simulink model "main_RI_LIEKF_GNSSOutrage"  (R2023a)
settings: Solver=FixedStepAuto  StartTime=0.0  StopTime=220  FixedStep=0.01  RelTol=1e-3
InitFcn:
  | initNavigation0612_AOA;
values from neighbouring files (symbols this model uses):
  CF_enable = 0    [initNavigation.m]
  dt = 0.01    [initNavigation.m]
  dtDelay = -0.03    [initNavigation.m]
  g0 = 9.795    [initNavigation.m]
  gam0_rad = 0/57.3    (= 0)    [initNavigation.m]
  GNSSoutragetime = 90    [initNavigation.m]
  H_sensor_type = 0    [initNavigation.m]
  KF_enable = 1    [initNavigation.m]
  P0 = diag([1*ones(3,1);0.01*ones(3,1);0.1*ones(3,1);0.001*ones(3,1);0.00001*ones(3,1)])    [initNavigation.m]
  P0_RIEKF = diag([1*ones(3,1);0.01*ones(3,1);0.1*ones(3,1);0.001*ones(3,1);0.00001*ones(3,1);      0.01*ones(3,1);[0;2;2]/57.3;[0.1;0.1;0.1]])^2    [initNavigation.m]
  pd0 = 0    [initNavigation.m]
  pe0 = 0    [initNavigation.m]
  phi0_rad = 0/57.3    (= 0)    [initNavigation.m]
  pn0 = 0    [initNavigation.m]
  psi = -178    [initNavigation.m]
  psi0_rad = 0/57.3    (= 0)    [initNavigation.m]
  state_dim = 24    [initNavigation.m]
  Time = 0:0.01:(size(traindata.AttackAngle,1) - 1)*0.01    [NNLiftCoefficientFit.m]
  vd0 = 0    [initNavigation.m]
  ve0 = 0    [initNavigation.m]
  vn0 = 0    [initNavigation.m]
undefined symbols (not defined in the file or in its folder): DiscIntNeverNeededParam, Discrete, INS_CONST, INS_EXPORT, INS_PARAM, magnitude, p, param, pInitialization, sys
libraries: simulink_extras x94, simulink x82, dspstat3 x70, sharedtransform x60, ctrlSharedLib x36, sharedTrackingLibrary x22, matrix_library x15, FMT_Model_Lib x13, deeplib x8, dspsolvers x4, vrlib x4, aerolibconvert2 x1
(part 25 of 28)

== matlab function main_RI_LIEKF_GNSSOutrage/State estimation/RI EKF_AOA_direct/Error State Kalman Filter/bak/Simulink Function - State Transition Jacobian/Cal Phi1/MATLAB Function1 ==
  data: vn input; Phi output; pn input; Rbn input; dt input
function Phi = fcn(vn,pn, Rbn,dt)
    
    %{
    F.block(0, 0, 3, 3) = exp_so3(-w_hat * dt);
        F.block(0, 9, 3, 3).noalias() = -exp_so3(-w_hat * dt) * Jr_so3(-w_hat * dt) * dt;
        F.block(9, 9, 3, 3).setIdentity();
        F.block(6, 0, 3, 3).noalias() = -R_Gtoi.transpose() * skew_x(a_hat * dt);
        F.block(6, 6, 3, 3).setIdentity();
        F.block(6, 12, 3, 3) = -R_Gtoi.transpose() * dt;
        F.block(12, 12, 3, 3).setIdentity();
        F.block(3, 0, 3, 3).noalias() = -0.5 * R_Gtoi.transpose() * skew_x(a_hat * dt * dt);
        F.block(3, 6, 3, 3) = Eigen::Matrix3d::Identity() * dt;
        F.block(3, 12, 3, 3) = -0.5 * R_Gtoi.transpose() * dt * dt;
        F.block(3, 3, 3, 3).setIdentity();
        Eigen::Matrix<double, 15, 12> G = Eigen::Matrix<double, 15, 12>::Zero();
    %}
    %
    %
    %F = [0_33         0_33  0_33   -Rbn          0_33]
    %    [skew(gn)     0_33  0_33  -skew(vn)Rbn   -Rbn]
    %    [0.5*skew(gn) I_33  0_33  -skew(pn)Rbn   -Rbn]
    %    [         0_69                  I66          ]
    Phi = zeros(15,15);
    g0 = 9.79;
    gn = [0;0;-g0];
    F  = zeros(15,15);
    F(1:3,10:12) = -Rbn;
    F(4:6,1:3)   = skewMat(gn);
    F(4:6,10:12) = -skewMat(vn)*Rbn;
    F(4:6,13:15) = -Rbn;
    F(7:9,4:6)   = eye(3);
    F(7:9,1:3)   = 0.5*skewMat(gn) * dt;
    F(7:9,10:12) = -skewMat(pn)*Rbn;
    F(7:9,13:15) = -Rbn;
    %F(10:15,10:15) = eye(6);
    Phi = eye(15) + F * dt;

end

== matlab function main_RI_LIEKF_GNSSOutrage/State estimation/RI EKF_AOA_direct/Error State Kalman Filter/bak/Simulink Function - State Transition Jacobian/MATLAB Function1 ==
  data: Rbn input; G output; vn input; pn input; dt input
function G = fcn(Rbn, vn,pn, dt)
    % G.block(0, 0, 3, 3) = -exp_so3(-w_hat * dt) * Jr_so3(-w_hat * dt) * dt;
    %    G.block(6, 3, 3, 3) = -R_Gtoi.transpose() * dt;
    %    G.block(3, 3, 3, 3) = -0.5 * R_Gtoi.transpose() * dt * dt;
    %    G.block(9, 6, 3, 3).setIdentity();
    %    G.block(12, 9, 3, 3).setIdentity();

    G = zeros(15,12);
    % G(1:3,1:3) = -  Rbn * dt;
    % G(4:6,1:3) = -skewMat(vn)*Rbn* dt;
    % G(4:6,4:6) =  - Rbn;
    % G(7:9,1:3) = -skewMat(pn)*Rbn * dt;
    % G(7:9,4:6) =  - Rbn;
    % G(10:12,7:9) = eye(3)*dt;
    % G(13:15,10:12) = eye(3)*dt;
    G(1:3,1:3) =  - Rbn * dt;
    G(4:6,1:3) = -skewMat(vn)*Rbn * dt;
    G(4:6,4:6) =  - Rbn* dt;
    G(7:9,1:3) = -skewMat(pn)*Rbn * dt;
    G(7:9,4:6) =  - Rbn* dt;
    G(10:12,7:9) = eye(3) ;
    G(13:15,10:12) = eye(3) ;
    
    %G = G*double(dt);
end

== matlab function main_RI_LIEKF_GNSSOutrage/State estimation/RI EKF_AOA_direct/INS propogation/AOA//SA//Vwind update/Subsystem/MATLAB Function ==
  data: u input; Rab output
function Rab = fcn(u)
    Rab = zeros(3,3);
        ca = cos(u(2));
        sa = sin(u(2));
        cb = cos(u(3));
        sb = sin(u(3));
    Rab = double([ca * cb,-ca * sb, -sa;
        sb, cb, 0;
        sa * cb, -sa * sb, ca;]);
end

== matlab function main_RI_LIEKF_GNSSOutrage/State estimation/RI EKF_AOA_direct/INS propogation/AOA//SA//Vwind update/Subsystem/MATLAB Function2 ==
  data: delta input; Rbn_correct output double size=[3,3]; Rbn input
function Rbn_correct = fcn(delta, Rbn)
    delta(1) = 0;
    Rbn_correct = zeros(3,3);
     %Rbn_correct = exp_so3(delta)* Rbn;
    Rbn_correct =double(( eye(3) + skewMat(delta))* Rbn);
end

== matlab function main_RI_LIEKF_GNSSOutrage/State estimation/RI EKF_AOA_direct/INS propogation/AOA//SA//Vwind update/Subsystem/Subsystem1/LSTM predict/MATLAB Function5 ==
  data: X input; X_nYPred output
function X_nYPred = LSTMnet(X)
    sig_X = [0.1167;0.1277;0.0579];
    sig_Y = 0.0451;
    mu_X = [0.0587;0.5185;-0.0515];
    mu_Y = 0.1011;
    X_norm = (X - mu_X) ./ sig_X;
    persistent X_nYPredorm_store;
    if isempty(X_nYPredorm_store)
        X_nYPredorm_store = zeros(1000,3);
    end

    X_nYPredorm_store = [X_nYPredorm_store(2:end,:);X_norm'];
    %[~,YPred_seq] = predictAndUpdateState(net.net,X_nYPredorm_store);
     X_nYPred = single(X_nYPredorm_store);
    % YPred_seq = predict(net.net,X_nYPredorm_store');
    % YPred_test = YPred_seq(end);
    % YPred_test = double(YPred_test* sig_Y + mu_Y)*57.3;

end

== matlab function main_RI_LIEKF_GNSSOutrage/State estimation/RI EKF_AOA_direct/INS propogation/AOA//SA//Vwind update/Subsystem/Subsystem1/LSTM predict/MATLAB Function6 ==
  data: YPred_test input; YPred_test_out output
function YPred_test_out = LSTMnet(YPred_test)
    sig_X = [0.1167;0.1277;0.0579];
    sig_Y = 0.0451;
    mu_X = [0.0587;0.5185;-0.0515];
    mu_Y = 0.1011;
    YPred_test_out = YPred_test(end);
    YPred_test_out = single(YPred_test_out* sig_Y + mu_Y)*57.3;

end

== matlab function main_RI_LIEKF_GNSSOutrage/State estimation/RI EKF_AOA_direct/INS propogation/AOA//SA//Vwind update/Subsystem/Subsystem1/LSTM predict1/MATLAB Function5 ==
  data: X input; X_nYPred output
function X_nYPred = LSTMnet(X)
    sig_X = [0.2380; 0.1523 ;0.0429;0.1379];
    sig_Y = 0.0690;
    mu_X = [0.0068;-0.0055;-0.0070;-0.0450];
    mu_Y = -0.0228;
    X_norm = (X - mu_X) ./ sig_X;
    persistent X_nYPredorm_store;
    if isempty(X_nYPredorm_store)
        X_nYPredorm_store = zeros(1000,4);
    end

    X_nYPredorm_store = [X_nYPredorm_store(2:end,:);X_norm'];
    %[~,YPred_seq] = predictAndUpdateState(net.net,X_nYPredorm_store);
     X_nYPred = single(X_nYPredorm_store);
    % YPred_seq = predict(net.net,X_nYPredorm_store');
    % YPred_test = YPred_seq(end);
    % YPred_test = double(YPred_test* sig_Y + mu_Y)*57.3;

end

== matlab function main_RI_LIEKF_GNSSOutrage/State estimation/RI EKF_AOA_direct/INS propogation/AOA//SA//Vwind update/Subsystem/Subsystem1/LSTM predict1/MATLAB Function6 ==
  data: YPred_test input; YPred_test_out output
function YPred_test_out = LSTMnet(YPred_test)
    sig_X = [0.2380; 0.1523 ;0.0429;0.1379];
    sig_Y = 0.0690;
    mu_X = [0.0068;-0.0055;-0.0070;-0.0450];
    mu_Y = -0.0228;
    YPred_test_out = YPred_test(end);
    YPred_test_out = single(YPred_test_out* sig_Y + mu_Y)*57.3;

end

== matlab function main_RI_LIEKF_GNSSOutrage/State estimation/RI EKF_AOA_direct/INS propogation/AOA//SA//Vwind update/Subsystem/Subsystem1/MATLAB Function1 ==
  data: axyz input; Cl output; TAS input; alpha input
function Cl = fcn(axyz, TAS,alpha)
ax = axyz(1);
az = axyz(3);
mess = 6.9;
g = 9.79;
rou = 1.225;
a = 1.4;
b = 0.36;
S = a*b;

q = 0.5 * rou * TAS^2;

azs = -ax * sin(alpha) + az * cos(alpha);
Cl = -mess * azs / (q * S);
end

== matlab function main_RI_LIEKF_GNSSOutrage/Sensor_Data_Process/IMU_Data_Process/accl_preprocessing2/MATLAB Function3 ==
  data: curr_input input; curr_output output single; sample_freq input; cutoff_freq input
function curr_output = second_LPF_Butter_x(curr_input,sample_freq,cutoff_freq)
   persistent input_x;
   persistent output_x;

   if isempty(input_x)
       input_x = [0;0;0];
   end
   
   if isempty(output_x)
       output_x = [0;0;0];
   end
    B = [0,0,0];
    A = [0,0,0];
    M_PI_F = 3.1415926;
	fr = sample_freq / cutoff_freq;
	ohm = tan( M_PI_F / fr );
	c = 1.0 + 2.0 * cos( M_PI_F / 4.0 ) * ohm + ohm * ohm;
	B(1) = ohm * ohm / c;
	B(2) = 2.0 * B(1);
	B(3) = B(1);
	A(1) = 2.0 * ( ohm * ohm - 1.0) / c;
	A(2) = (1.0 - 2.0 * cos( M_PI_F / 4.0 ) * ohm + ohm * ohm) / c;
	%/*获取最新输入*/
	input_x(3) = curr_input;
	%/* Butterworth */
	output_x(3) =B(1) * input_x(3) + B(2) * input_x(2) +B(3) * input_x(1) - A(1) * output_x(2) - A(2) * output_x(1);
	curr_output = single(output_x(3));
   % /* 输入序列保存 */
	input_x(1) = input_x(2);
	input_x(2) = input_x(3);
	%/*输出序列保存 */
	output_x(1) = output_x(2);
	output_x(2) = output_x(3);

== matlab function main_RI_LIEKF_GNSSOutrage/State estimation/RI EKF_AOA_direct/INS propogation/AOA//SA//Vwind update/Subsystem/Subsystem1/MATLAB Function3 ==
  data: axyz input; Cy output; TAS input; alpha input; beta input
function Cy = fcn(axyz, TAS,alpha,beta)
ax = axyz(1);
ay = axyz(2);
az = axyz(3);

mess = 6.9;
g = 9.79;
rou = 1.225;
a = 1.4;
b = 0.36;
S = a*b;

q = 0.5 * rou * TAS^2;
ays = -ax .* cos(alpha).*sin(beta) + ay .* cos(beta) - az .* sin(alpha).* sin(beta);
% azs = -ax * sin(alpha) + az * cos(alpha);
Cy = mess * ays / (q * S);
end

== matlab function main_RI_LIEKF_GNSSOutrage/State estimation/RI EKF_AOA_direct/INS propogation/AOA//SA//Vwind update/Subsystem/Subsystem1/MATLAB Function4 ==
  data: u input; CalculatedAttackAngleFiltered output
function CalculatedAttackAngleFiltered = fcn(u)
PitchRate = u(1);
cl = u(2);
ElevatorAngle = u(3);

coefficients_filtered = [0.0236, -0.4283, -0.0765, -0.0898];

    
CalculatedAttackAngleFiltered = (cl - ...
    coefficients_filtered(1) - ...
    coefficients_filtered(3) * PitchRate - ...
    coefficients_filtered(4) * ElevatorAngle) / coefficients_filtered(2);


end

== matlab function main_RI_LIEKF_GNSSOutrage/State estimation/RI EKF_AOA_direct/INS propogation/att update/MATLAB Function ==
  data: Rbn_k_1 input; Rbn output; w input; dt input
function Rbn = fcn(Rbn_k_1, w, dt)
    Rbn =  Rbn_k_1 * exp_so3( w * dt);
end

== matlab function main_RI_LIEKF_GNSSOutrage/State estimation/RI EKF_AOA_direct/INS propogation/att update/MATLAB Function2 ==
  data: delta input; Rbn_correct output single size=[3,3]; Rbn input
function Rbn_correct = fcn(delta, Rbn)
    Rbn_correct = zeros(3,3);
     Rbn_correct = exp_so3(delta)* Rbn;
    %Rbn_correct =( eye(3) + skewMat(delta))* Rbn;
end

== matlab function main_RI_LIEKF_GNSSOutrage/State estimation/RI EKF_AOA_direct/INS propogation/vel//pos update/pos update/MATLAB Function ==
  data: dtheta input; pos_correct output single; KFState_dp input; pos input
function pos_correct = fcn(dtheta, KFState_dp, pos)
    
     pos_correct =  KFState_dp + exp_so3(dtheta)*pos;
    %pos_correct = pos + KFState_dp - skewMat(pos)*dtheta;
    
end

== matlab function main_RI_LIEKF_GNSSOutrage/State estimation/RI EKF_AOA_direct/INS propogation/vel//pos update/vel update/MATLAB Function ==
  data: dtheta input; vel_correct output single; KFState_dv input; vel input
function vel_correct = fcn(dtheta, KFState_dv, vel)
    
     vel_correct =  KFState_dv + exp_so3( dtheta)*vel;
    %vel_correct =  vel + KFState_dv - skewMat(vel)*dtheta;
end

== matlab function main_RI_LIEKF_GNSSOutrage/State estimation/LI EKF2/Error State Kalman Filter/Extended Kalman Filter1/Correct1/IGG_check/MATLAB Function ==
  data: err input; w output; k0 input; k1 input; zk0 input; zk1 input
function w = fcn(err,k0,k1,zk0,zk1)
    err = abs(err);  w = err;
    for k=1:2
        if err(k)<=k0,    w(k)=1;
        elseif err(k)>k1, w(k)=0;
        else,             w(k)=k0/err(k);  
        end
    end
        if err(3)<=zk0,    w(3)=1;
        elseif err(3)>zk1, w(3)=0;
        else,             w(3)=zk0/err(3);  
        end
end

== matlab function main_RI_LIEKF_GNSSOutrage/State estimation/LI EKF2/Error State Kalman Filter/Extended Kalman Filter1/Output/MATLAB Function ==
  data: S input; P output
function P = fcn(S)
    
    % Get back Covariance from Square-root Covariance
    P = S*S';
    
end

== matlab function main_RI_LIEKF_GNSSOutrage/State estimation/LI EKF2/Error State Kalman Filter/Extended Kalman Filter1/Predict/Predict ==
  settings: updateMethod=DISCRETE  sampleTime=SampleTime
  data: x input; xNew output; P input; Q input; uState input; unused input; P output; pS parameter
function [xNew,P] = fcn(x,P,Q,uState,~,pS)
% ekfCorrect Prediction step for EKF
%
%   Copyright 2016-2021 The MathWorks, Inc.

%#codegen

% If process noise is time-varying then compute square-root
% factorization.
if pS.HasTimeVaryingQ
   Q = matlabshared.tracking.internal.svdPSD(Q);
end

% Construct fcn handles
if pS.IsSimulinkFcn
    StateTransitionJacobianFcnH_SL = str2func(pS.FcnName);
    if pS.HasAdditiveNoise
        StateTransitionFcnH = @(fState)StateTransitionJacobianFcnH_SL(fState);
    else
        StateTransitionFcnH = @(fState,fProcNoise)StateTransitionJacobianFcnH_SL(fState,fProcNoise);
    end
else
    StateTransitionFcnH = str2func(pS.FcnName);
end
if pS.HasJacobian
    if pS.IsSimulinkFcn
        StateTransitionJacobianFcnH_SL = str2func(pS.JacobianFcnName);
        if pS.HasAdditiveNoise
            StateTransitionJacobianFcnH = @(fState)StateTransitionJacobianFcnH_SL(fState);
        else
            StateTransitionJacobianFcnH = @(fState,fProcNoise)StateTransitionJacobianFcnH_SL(fState,fProcNoise);
        end
    else
        StateTransitionJacobianFcnH = str2func(pS.JacobianFcnName);
    end
else
    StateTransitionJacobianFcnH = [];
end

switch pS.NumberOfExtraArgumentInports
    case 0
        extraArgs = {};
    case 1
        extraArgs = {uState};
    otherwise
        assert(false);
end

% Check if dimensions and type of State and Jacobian are correct
if pS.HasAdditiveNoise
   % Additive noise
   
   % StateTransitionFcn
   xTry = StateTransitionFcnH(x, extraArgs{:});
   
   if pS.IsSimulinkFcn
      hasError = any(size(x) ~= size(xTry));
   else
      hasError = any(size(x) ~= size(xTry)) || ~isa(xTry, class(x));
   end
   
   coder.internal.errorIf(...
      hasError,...
      'shared_tracking:ExtendedKalmanFilter:StateNonMatchingSizeOrClass',...
      'StateTransitionFcn', 'State', numel(x));
   
   if pS.HasJacobian
      % Jacobian
      F = StateTransitionJacobianFcnH(x, extraArgs{:});
      % F needs to be square
      isSizeNotCorrect = ~all(size(F) == numel(x));
      
      if pS.IsSimulinkFcn
         hasError = isSizeNotCorrect;
      else
         hasError = isSizeNotCorrect || ~isa(F, class(x));
      end
      
      coder.internal.errorIf(...
         hasError,...
         'shared_tracking:ExtendedKalmanFilter:StateTransitionJacobianNonMatchingSizeOrClass',...
         'StateTransitionJacobianFcn', numel(x));
   end
else
   % Non-additive noise
   
   % StateTransitionFcn
   xTry = StateTransitionFcnH(x, zeros(size(Q,1),1,'like',x),extraArgs{:});
   
   if pS.IsSimulinkFcn
      hasError = any(size(x) ~= size(xTry));
   else
      hasError = any(size(x) ~= size(xTry)) || ~isa(xTry, class(x));
   end
   
   coder.internal.errorIf(...
      hasError,...
      'shared_tracking:ExtendedKalmanFilter:StateNonMatchingSizeOrClass',...
      'StateTransitionFcn', 'State', numel(x))
   
   if pS.HasJacobian
      % Jacobian
      F = StateTransitionJacobianFcnH(x, zeros(size(Q,1),1,'like',x),extraArgs{:});
      % F needs to be square
      isSizeNotCorrect = ~all(size(F) == numel(x));
      
      if pS.IsSimulinkFcn
         hasError = isSizeNotCorrect;
      else
         hasError = isSizeNotCorrect || ~isa(F, class(x));
      end
       
      coder.internal.errorIf(...
         hasError,...
         'shared_tracking:ExtendedKalmanFilter:StateTransitionJacobianNonMatchingSizeOrClass',...
         'StateTransitionJacobianFcn', numel(x));
   end
end

xNew = zeros(size(x),'like',x); %#ok<PREALL>

if pS.HasAdditiveNoise
    [xNew,P] = matlabshared.tracking.internal.EKFPredictorAdditive.predict(...
        Q,x,P,StateTransitionFcnH,StateTransitionJacobianFcnH,extraArgs{:});
else    
    [xNew,P] = matlabshared.tracking.internal.EKFPredictorNonAdditive.predict(...
        Q,x,P,StateTransitionFcnH,StateTransitionJacobianFcnH,extraArgs{:});
end
end

== matlab function main_RI_LIEKF_GNSSOutrage/State estimation/LI EKF2/Error State Kalman Filter/MATLAB Function ==
  data: u input; dp output size=3; dv output size=3; dtheta output size=3; da output size=3; dg output size=3; dm output size=3; dtheta_a output size=3; dv_wind output size=3
function [dp,dv,dtheta,da,dg,dm,dtheta_a,dv_wind] = fcn(u)
    dtheta = u(1:3);
    dv = u(4:6);
    dp = u(7:9);
    dg = u(10:12);
    da = u(13:15);
    dm = u(16:18);
    dtheta_a = u(19:21);
    dv_wind = u(22:24);
end

== matlab function main_RI_LIEKF_GNSSOutrage/Subsystem2/MATLAB Function1 ==
  data: x input; angleHeadingAB0to360 output
function angleHeadingAB0to360 = fcn(x)
 x = x -180;


    if  x >= 0 && x < 90           %第一象限，范围 [0,90)deg，0度应该会出现
        angleHeadingAB0to360  =   x;
    elseif x >= 90 && x < 180       %第二象限，范围 [90,180)deg
        angleHeadingAB0to360 = x;
    elseif x >= 180 && x < 270     %第三象限，范围 [180,270)deg，180度也应该会出现
        angleHeadingAB0to360 = - 360 + x;
    elseif x >= 270 && x < 360      %第四象限，范围 [270,360)deg
        angleHeadingAB0to360  = - 360+x;
    elseif x< 0 && x>-90 
        angleHeadingAB0to360  =   x;
    elseif x<= -90 && x>-180
        angleHeadingAB0to360  =   x;
    elseif x <= -180 && x >= -360
        angleHeadingAB0to360  =   x + 360;
    elseif x == 0 && x == 360 
        angleHeadingAB0to360 =single(0);
    else
         angleHeadingAB0to360  =   x;
    end
end

== matlab function main_RI_LIEKF_GNSSOutrage/State estimation/distribute CF/distribute CF/Correct/Attitude_Correction/Attitude_Correct/Subsystem2/MATLAB Function ==
  data: abs_v input; y output; gps_acc input
function y = fcn(abs_v,gps_acc)
if abs_v < 0.1
    y = double(zeros(3,1));
elseif abs_v  >= 0.1 && abs_v < 1
    y = double(0.7* gps_acc);
else
    y = double(1 * gps_acc);
end

== matlab function main_RI_LIEKF_GNSSOutrage/State estimation/distribute CF/distribute CF/Update/Attitude_Update/QuatMult1 ==
  data: quatA input; quatOut output single; quatB input
function quatOut = QuatMult(quatA,quatB)
% Calculate the following quaternion product quatA * quatB using the 
% standard identity 

quatOut = [quatA(1)*quatB(1)-quatA(2:4)'*quatB(2:4); quatA(1)*quatB(2:4) + quatB(1)*quatA(2:4) + cross(quatA(2:4),quatB(2:4))];

== matlab function main_RI_LIEKF_GNSSOutrage/State estimation/distribute CF/distribute CF/Update/Attitude_Update/rv2q ==
  data: rotVec input single; quaternion output single
% convert froma rotation vector in radians to a quaternion
function quaternion = RotToQuat(rotVec)

vecLength = sqrt(rotVec(1)^2 + rotVec(2)^2 + rotVec(3)^2);

if vecLength < 1e-6
  quaternion = single([1;0;0;0]);
else
  quaternion = single([cos(0.5*vecLength); rotVec/vecLength*sin(0.5*vecLength)]);
end

== matlab function main_RI_LIEKF_GNSSOutrage/State estimation/LI EKF2/Error State Kalman Filter/Simulink Function - GPS Measurements/MATLAB Function ==
  data: vn input; H output; pn input
function H = fcn(vn, pn)
    state_dim = 24;
    H = zeros(6,state_dim);
    % H(1:3,1:3) = skewMat(vn);
    % H(4:6,1:3) = skewMat(pn);
    H(1:6,4:9) = eye(6);
    %H = -H;
end

== matlab function main_RI_LIEKF_GNSSOutrage/State estimation/LI EKF2/Error State Kalman Filter/Simulink Function - GPS Measurements/MATLAB Function1 ==
  data: Rbn input; vn input; X_inv output; pn input
function X_inv = invX(Rbn, vn, pn)
    X_inv = zeros(5,5);
    Rnb = Rbn';
    X_inv(1:3,1:3) = Rnb;
    X_inv(1:3,4) = -Rnb * vn;
    X_inv(1:3,5) = -Rnb * pn;
    X_inv(4:5,4:5) = eye(2);
end

== matlab function main_RI_LIEKF_GNSSOutrage/State estimation/LI EKF2/Error State Kalman Filter/Simulink Function - GPS Measurements1/MATLAB Function ==
  data: vn input; H_baro output; pn input
function H_baro = fcn(vn, pn)
    state_dim = 24;
    H = zeros(6,state_dim);
    H(1:3,1:3) = skewMat(vn);
    H(4:6,1:3) = skewMat(pn);
    H(1:6,4:9) = eye(6);
    
    A = [0 0 0 0 0 1];
    H_baro = A * H;
end

== matlab function main_RI_LIEKF_GNSSOutrage/State estimation/LI EKF2/Error State Kalman Filter/Simulink Function - GPS Measurements2/MATLAB Function ==
  data: Rbn input; Magn input; H output; dtheta input
function H = fcn(Rbn, Magn, dtheta)
    state_dim = 24;
    H = zeros(3,state_dim);
    H(1:3,1:3) =  Rbn * skewMat(Magn);
    H(1:3,16:18) =  Rbn * skewMat(dtheta);
end

== matlab function main_RI_LIEKF_GNSSOutrage/State estimation/LI EKF2/Error State Kalman Filter/Simulink Function - GPS Measurements3/MATLAB Function ==
  data: Rbn input; Rab input; H output; vn input; v_wind input
function H = fcn(Rbn,Rab, vn,v_wind)
    state_dim = 24;
    A = Rab' * Rbn';
    H = zeros(3,state_dim);
   % H(1:3,1:3) =  - skewMat(vn - v_wind);
   % H(1:3,4:6) =  eye(3);
    H(1:3,19:21) =  - skewMat(vn - v_wind);
    H(1:3,22:24) =  - eye(3);
    H = double(A * H);
end

== matlab function main_RI_LIEKF_GNSSOutrage/State estimation/bak1/Error State Kalman Filter/Extended Kalman Filter1/Correct1/Correct ==
  settings: updateMethod=DISCRETE  sampleTime=SampleTime
  data: x input; xNew output; P input; P output; yMeas input; R input; uMeas input; blockOrdering input; pM parameter; blockOrdering output
function [xNew,P,blockOrdering] = fcn(x,P,yMeas,R,uMeas,blockOrdering,pM)
% ekfCorrect Correction step for EKF
%
%   Copyright 2016-2021 The MathWorks, Inc.

%#codegen

% If measurement noise is time-varying then compute square-root
% factorization.
if pM.HasTimeVaryingR
   R = matlabshared.tracking.internal.svdPSD(R);
end

% Construct the function handle for measurement fcn
if pM.IsSimulinkFcn
    MeasurementFcnH_SL = str2func(pM.FcnName);
    if pM.HasAdditiveNoise
        MeasurementFcnH = @(fState)MeasurementFcnH_SL(fState);
    else
        MeasurementFcnH = @(fState,fMeasNoise)MeasurementFcnH_SL(fState,fMeasNoise);
    end
else
    MeasurementFcnH = str2func(pM.FcnName);
end

% Construct the function handle for measurement Jacobian fcn
if pM.HasJacobian
    if pM.IsSimulinkFcn
        MeasurementJacobianFcnH_SL = str2func(pM.JacobianFcnName);
        if pM.HasAdditiveNoise
            MeasurementJacobianFcnH = @(fState)MeasurementJacobianFcnH_SL(fState);
        else
            MeasurementJacobianFcnH = @(fState,fMeasNoise)MeasurementJacobianFcnH_SL(fState,fMeasNoise);
        end
    else
        MeasurementJacobianFcnH = str2func(pM.JacobianFcnName);
    end
else
    MeasurementJacobianFcnH = [];
end

% Handle (optional) extra input arguments of the measurement & jacobian fcns
switch pM.NumberOfExtraArgumentInports
    case 0
        extraArgs = {};
    case 1
        extraArgs = {uMeas};
    otherwise
        assert(false);
end

% Construct the corrector, perform the update
if pM.HasAdditiveNoise
    ekfCorrector = matlabshared.tracking.internal.EKFCorrectorAdditive();
else
    ekfCorrector = matlabshared.tracking.internal.EKFCorrectorNonAdditive();
end

% Check if dimensions and type of Measurement and Jacobian are correct
if pM.HasAdditiveNoise
   % Additive noise
   
   % MeasurementFcn
   ztry = MeasurementFcnH(x, extraArgs{:});
   
   if pM.IsSimulinkFcn
      hasError = (numel(ztry) ~= numel(yMeas));
   else
      hasError = (numel(ztry) ~= numel(yMeas)) || ~isa(ztry, class(x));
   end
   
   coder.internal.errorIf(...
      hasError,...
      'shared_tracking:ExtendedKalmanFilter:MeasurementNonMatchingSizeOrClass',...
      'MeasurementFcn');
   
   if pM.HasJacobian
      % MeasurementJacobianFcn
      Htry = MeasurementJacobianFcnH(x, extraArgs{:});
      isSizeNotCorrect = numel(yMeas) ~= size(Htry,1) || numel(x) ~= size(Htry,2);
      
      if pM.IsSimulinkFcn
         hasError = isSizeNotCorrect;
      else
         hasError = isSizeNotCorrect || ~isa(Htry, class(x));
      end
      
      coder.internal.errorIf(...
         hasError,...
         'shared_tracking:ExtendedKalmanFilter:MeasurementJacobianNonMatchingSizeOrClass',...
         'MeasurementJacobianFcn',numel(yMeas),numel(x));
   end   
else
   % Non-additive noise
   
   % MeasurementFcn
   ztry = MeasurementFcnH(...
      x, zeros(size(R,1),1,'like',x), ...
      extraArgs{:});   

   if pM.IsSimulinkFcn
      hasError = (numel(ztry) ~= numel(yMeas));
   else
      hasError = (numel(ztry) ~= numel(yMeas)) || ~isa(ztry, class(x));
   end
   
   coder.internal.errorIf(...
      hasError,...
      'shared_tracking:ExtendedKalmanFilter:MeasurementNonMatchingSizeOrClass',...
      'MeasurementFcn');
   
   if pM.HasJacobian
      % MeasurementJacobianFcn
      Htry = MeasurementJacobianFcnH(...
         x, zeros(size(R,1),1,'like',x), ...
         extraArgs{:});
      
      isSizeNotCorrect = numel(yMeas) ~= size(Htry,1) || numel(x) ~= size(Htry,2);     
      
      if pM.IsSimulinkFcn
         hasError = isSizeNotCorrect;
      else
         hasError = isSizeNotCorrect || ~isa(Htry, class(x));
      end
      
      coder.internal.errorIf(...
         hasError,...
         'shared_tracking:ExtendedKalmanFilter:MeasurementJacobianNonMatchingSizeOrClass',...
         'MeasurementJacobianFcn',numel(yMeas),numel(x));
   end
end
% Measurement wrapping
ekfCorrector.HasMeasurementWrapping = pM.HasWrapping;

xNew = zeros(size(x),'like',x); %#ok<PREALL>
% wk = 0;
[xNew,P] = ekfCorrector.correct(...
        yMeas,R,x,P,MeasurementFcnH,MeasurementJacobianFcnH,extraArgs{:});
end

== matlab function main_RI_LIEKF_GNSSOutrage/State estimation/LI EKF2/Error State Kalman Filter/Simulink Function - State Transition/Cal Phi/MATLAB Function2 ==
  data: w input; Phi output; a input; Rbn input; dt input
function Phi = fcn(w,a, Rbn,dt)
    Phi = cal_LIEKF_F(w,a, Rbn,dt);

end

== matlab function main_RI_LIEKF_GNSSOutrage/State estimation/LI EKF2/Error State Kalman Filter/Simulink Function - State Transition/MATLAB Function1 ==
  data: Rbn input; G output; dt input
function G = fcn(Rbn, dt)
       G = cal_LIEKF_G(Rbn, dt);

end

== matlab function main_RI_LIEKF_GNSSOutrage/State estimation/LI EKF2/Error State Kalman Filter/Simulink Function - State Transition1/Cal Phi/MATLAB Function1 ==
  data: w input; Phi output; a input; Rbn input; dt input
function Phi = fcn(w,a, Rbn,dt)
    Phi = cal_LIEKF_F(w,a, Rbn,dt);
end

== matlab function main_RI_LIEKF_GNSSOutrage/State estimation/LI EKF2/Error State Kalman Filter/Simulink Function - State Transition1/MATLAB Function1 ==
  data: Rbn input; G output; dt input
function G = fcn(Rbn, dt)
   G = cal_LIEKF_G(Rbn, dt);
end

== matlab function main_RI_LIEKF_GNSSOutrage/State estimation/LI EKF2/Error State Kalman Filter/bak/MATLAB Function1 ==
  data: Cbn input; wxyz input; ZeroVelDetectFlag output; fbxyz input; fex input; ZeroVelDetectFlagold output
function [ZeroVelDetectFlag,ZeroVelDetectFlagold]  = ZeroVelDetect(Cbn, wxyz,fbxyz, fex)
%% Use buffer to restore IMU data
    Windows = 8;
    tao = 0.8;
    ZeroVelDetectFlag = false;
    ZeroVelDetectFlagold = false;
    persistent w_;
    persistent a_;
    
    if isempty(w_) && isempty(a_)
        w_ = single(zeros(3,Windows));
        a_ = single(zeros(3,Windows));
    end
    w_ = [w_(:,2:Windows),wxyz];
    a_ = [a_(:,2:Windows),fbxyz];
    
    g=9.79;

    sigma2_a = 0.009^2;
    sigma2_g = 0.025^2;
    %sigma2_fex = 0.01^2;
    T = single(0);
    T_old = single(0);
    
    ya_m=mean(a_,2);
    for k=Windows-1
         tmp_old=a_(:,k)-g*ya_m/norm(ya_m);
        
        T_old = T_old + w_(:,k)'*w_(:,k)/sigma2_g+tmp_old'*tmp_old/sigma2_a;
        T = T + w_(:,k)'*w_(:,k)/sigma2_g;
        T_old = T_old + w_(:,k)'*w_(:,k)/sigma2_g;
    end
    T=T/Windows;
    T_old=T_old/Windows;
    T_fex = (fex + Cbn'*[0;0;g])'*(fex + Cbn'*[0;0;g]);
    T = T + T_fex;
    w = w_;
    a = a_;

    if T < tao 
        ZeroVelDetectFlag = true;
    end
    if T_old < tao 
        ZeroVelDetectFlagold = true;
    end
end

== matlab function main_RI_LIEKF_GNSSOutrage/State estimation/LI EKF2/Error State Kalman Filter/bak/RIEKF ==
  data: Rbn input; vn input; pn input; bg input; ba input; phi input; Q input; P input; dt input; GNSS_Mea input; GNSS_flag input; Rbn_update output; vn_update output; pn_update output; bg_update output; ba_update output; cov output
function [Rbn_update,vn_update,pn_update,bg_update,ba_update,cov] = RIEKF(Rbn,vn,pn,bg,ba,phi,Q,P,dt,GNSS_Mea,GNSS_flag)
    %initial state
    state.Rbn = Rbn;
    state.vn = vn;
    state.pn = pn;
    state.bg = bg;
    state.ba = ba;
    state = Construct_State(state);
    %initial RIEKF filter 
    RIEKF.P = P;
    RIEKF.phi = phi;
%% Error State Predict
    RIEKF.Qk = RIEKF.phi * Q * RIEKF.phi' * dt;             %Qk = φ·Q·φ·δt
    RIEKF.P = RIEKF.phi * RIEKF.P * RIEKF.phi' + RIEKF.Qk;  %P = φ·P·φ + Qk
    RIEKF.H_GNSS = calH(state.vn, state.pn);                %H
    RIEKF.Y = GNSS_Mea;
    RIEKF.b_GNSS = [zeros(1,2);eye(2)]; %    [0 0]
                                        %b = [1 0]
                                        %    [0 1]
    RIEKF.noise_GNSS = diag([0.01*ones(3,1);0.01*ones(3,1)]); %set GNSS error conv
%%
    if (GNSS_flag == 1)
        [state,RIEKF] = GNSSupdate(state,RIEKF);
    end
    Rbn_update = state.Rbn;
    vn_update = state.vn;
    pn_update = state.pn;
    bg_update = state.bg;
    ba_update = state.ba;
    cov = RIEKF.P;
end

function state = Construct_State(state)
            state.X = zeros(5,5);
            state.X(1:5,1:5) = [state.Rbn, state.vn, state.pn; 
                            zeros(1,3),1,0; 
                            zeros(1,3),0,1;];
            % Add Landmarks
            % Parameters
           state.bias = [state.bg; state.ba];
end

function [state,RIEKF] = GNSSupdate(state,RIEKF)
    % correct
    S = RIEKF.H_GNSS  * RIEKF.P * RIEKF.H_GNSS' + RIEKF.noise_GNSS; %噪声R矩阵的处理是否需要变换？
    K = (RIEKF.P * RIEKF.H_GNSS')/S;
    innonation = state.X * RIEKF.Y - RIEKF.b_GNSS;

    delta = K * innonation;
    dX = expMat(delta(1:end-6));
    dbias = delta(end-5:end);
    state.X = dX * state.X;
    state.bias = state.bias + dbias;
    state = updatestate(state);
    I = eye(size(RIEKF.P));
    RIEKF.P = (I - K*RIEKF.H_GNSS )* RIEKF.P *(I - K*RIEKF.H_GNSS )' + K*RIEKF.noise_GNSS*K';
end

function eX = expMat(delta)
    eX = zeros(5,5);
    eX(1:3,1:3) = exp_so3(delta(1:3));
    eX(1:3,4) = reshape(delta(4:6),3,1);
    eX(1:3,5) = reshape(delta(7:9),3,1);
    eX(4,4) = 1;
    eX(5,5) = 1;
end

function R = exp_so3(w)
    w_x  = [0, -w(3), w(2);
            w(3), 0, -w(1);
            -w(2), w(1), 0];
    theta = norm(w);
    if theta < 1e-7
        A = 1;
        B = 0.5;
    else
        A = double(sin(theta) / theta);
        B = double((1 - cos(theta)) / (theta * theta));
    end
    
    if theta == 0
        R = double(eye(3));
    else
        R = double(eye(3) + A * w_x + B * w_x * w_x);
    end
end

function H = calH(vn, pn)
    H = zeros(6,15);
    H(1:3,1:3) = -skewMat(vn);
    H(4:6,1:3) = -skewMat(pn);
    H(1:6,4:9) = eye(6);
end

function state = updatestate(state)
        state.Rbn = state.X(1:3,1:3);
        state.vn = state.X(1:3,4);
        state.pn = state.X(1:3,5);
        state.bg = state.bias(1:3);
        state.ba = state.bias(4:6);
end

== matlab function main_RI_LIEKF_GNSSOutrage/State estimation/LI EKF2/Error State Kalman Filter/bak/Simulink Function - GPS Measurements1/MATLAB Function1 ==
  data: H output; Cbn input; dt input
function H = calH(Cbn, dt)
    

    H = zeros(3,18);
    % 

    H(1:3,4:6) = eye(3);
    H(1:3,16:18) = -Cbn * dt;
end

== matlab function main_RI_LIEKF_GNSSOutrage/State estimation/LI EKF2/Error State Kalman Filter/bak/Simulink Function - State Transition Jacobian/Cal Phi1/MATLAB Function1 ==
  data: vn input; Phi output; pn input; Rbn input; dt input
function Phi = fcn(vn,pn, Rbn,dt)
    
    %{
    F.block(0, 0, 3, 3) = exp_so3(-w_hat * dt);
        F.block(0, 9, 3, 3).noalias() = -exp_so3(-w_hat * dt) * Jr_so3(-w_hat * dt) * dt;
        F.block(9, 9, 3, 3).setIdentity();
        F.block(6, 0, 3, 3).noalias() = -R_Gtoi.transpose() * skew_x(a_hat * dt);
        F.block(6, 6, 3, 3).setIdentity();
        F.block(6, 12, 3, 3) = -R_Gtoi.transpose() * dt;
        F.block(12, 12, 3, 3).setIdentity();
        F.block(3, 0, 3, 3).noalias() = -0.5 * R_Gtoi.transpose() * skew_x(a_hat * dt * dt);
        F.block(3, 6, 3, 3) = Eigen::Matrix3d::Identity() * dt;
        F.block(3, 12, 3, 3) = -0.5 * R_Gtoi.transpose() * dt * dt;
        F.block(3, 3, 3, 3).setIdentity();
        Eigen::Matrix<double, 15, 12> G = Eigen::Matrix<double, 15, 12>::Zero();
    %}
    %
    %
    %F = [0_33         0_33  0_33   -Rbn          0_33]
    %    [skew(gn)     0_33  0_33  -skew(vn)Rbn   -Rbn]
    %    [0.5*skew(gn) I_33  0_33  -skew(pn)Rbn   -Rbn]
    %    [         0_69                  I66          ]
    Phi = zeros(15,15);
    g0 = 9.79;
    gn = [0;0;-g0];
    F  = zeros(15,15);
    F(1:3,10:12) = -Rbn;
    F(4:6,1:3)   = skewMat(gn);
    F(4:6,10:12) = -skewMat(vn)*Rbn;
    F(4:6,13:15) = -Rbn;
    F(7:9,4:6)   = eye(3);
    F(7:9,1:3)   = 0.5*skewMat(gn) * dt;
    F(7:9,10:12) = -skewMat(pn)*Rbn;
    F(7:9,13:15) = -Rbn;
    %F(10:15,10:15) = eye(6);
    Phi = eye(15) + F * dt;

end

== matlab function main_RI_LIEKF_GNSSOutrage/State estimation/LI EKF2/Error State Kalman Filter/bak/Simulink Function - State Transition Jacobian/MATLAB Function1 ==
  data: Rbn input; G output; vn input; pn input; dt input
function G = fcn(Rbn, vn,pn, dt)
    % G.block(0, 0, 3, 3) = -exp_so3(-w_hat * dt) * Jr_so3(-w_hat * dt) * dt;
    %    G.block(6, 3, 3, 3) = -R_Gtoi.transpose() * dt;
    %    G.block(3, 3, 3, 3) = -0.5 * R_Gtoi.transpose() * dt * dt;
    %    G.block(9, 6, 3, 3).setIdentity();
    %    G.block(12, 9, 3, 3).setIdentity();

    G = zeros(15,12);
    % G(1:3,1:3) = -  Rbn * dt;
    % G(4:6,1:3) = -skewMat(vn)*Rbn* dt;
    % G(4:6,4:6) =  - Rbn;
    % G(7:9,1:3) = -skewMat(pn)*Rbn * dt;
    % G(7:9,4:6) =  - Rbn;
    % G(10:12,7:9) = eye(3)*dt;
    % G(13:15,10:12) = eye(3)*dt;
    G(1:3,1:3) =  - Rbn * dt;
    G(4:6,1:3) = -skewMat(vn)*Rbn * dt;
    G(4:6,4:6) =  - Rbn* dt;
    G(7:9,1:3) = -skewMat(pn)*Rbn * dt;
    G(7:9,4:6) =  - Rbn* dt;
    G(10:12,7:9) = eye(3) ;
    G(13:15,10:12) = eye(3) ;
    
    %G = G*double(dt);
end

== matlab function main_RI_LIEKF_GNSSOutrage/State estimation/LI EKF2/INS propogation/AOA//SA//Vwind update/Subsystem/LSTM predict/MATLAB Function5 ==
  data: X input; X_nYPred output
function X_nYPred = LSTMnet(X)
    sig_X = [0.1167;0.1277;0.0579];
    sig_Y = 0.0451;
    mu_X = [0.0587;0.5185;-0.0515];
    mu_Y = 0.1011;
    X_norm = (X - mu_X) ./ sig_X;
    persistent X_nYPredorm_store;
    if isempty(X_nYPredorm_store)
        X_nYPredorm_store = zeros(1000,3);
    end

    X_nYPredorm_store = [X_nYPredorm_store(2:end,:);X_norm'];
    %[~,YPred_seq] = predictAndUpdateState(net.net,X_nYPredorm_store);
     X_nYPred = single(X_nYPredorm_store);
    % YPred_seq = predict(net.net,X_nYPredorm_store');
    % YPred_test = YPred_seq(end);
    % YPred_test = double(YPred_test* sig_Y + mu_Y)*57.3;

end

== matlab function main_RI_LIEKF_GNSSOutrage/State estimation/LI EKF2/INS propogation/AOA//SA//Vwind update/Subsystem/LSTM predict/MATLAB Function6 ==
  data: YPred_test input; YPred_test_out output
function YPred_test_out = LSTMnet(YPred_test)
    sig_X = [0.1167;0.1277;0.0579];
    sig_Y = 0.0451;
    mu_X = [0.0587;0.5185;-0.0515];
    mu_Y = 0.1011;
    YPred_test_out = YPred_test(end);
    YPred_test_out = single(YPred_test_out* sig_Y + mu_Y)*57.3;

end

== matlab function main_RI_LIEKF_GNSSOutrage/State estimation/LI EKF2/INS propogation/AOA//SA//Vwind update/Subsystem/LSTM predict1/MATLAB Function5 ==
  data: X input; X_nYPred output
function X_nYPred = LSTMnet(X)
    sig_X = [0.2380; 0.1523 ;0.0429;0.1379];
    sig_Y = 0.0690;
    mu_X = [0.0068;-0.0055;-0.0070;-0.0450];
    mu_Y = -0.0228;
    X_norm = (X - mu_X) ./ sig_X;
    persistent X_nYPredorm_store;
    if isempty(X_nYPredorm_store)
        X_nYPredorm_store = zeros(1000,4);
    end

    X_nYPredorm_store = [X_nYPredorm_store(2:end,:);X_norm'];
    %[~,YPred_seq] = predictAndUpdateState(net.net,X_nYPredorm_store);
     X_nYPred = single(X_nYPredorm_store);
    % YPred_seq = predict(net.net,X_nYPredorm_store');
    % YPred_test = YPred_seq(end);
    % YPred_test = double(YPred_test* sig_Y + mu_Y)*57.3;

end

== matlab function main_RI_LIEKF_GNSSOutrage/State estimation/LI EKF2/INS propogation/AOA//SA//Vwind update/Subsystem/LSTM predict1/MATLAB Function6 ==
  data: YPred_test input; YPred_test_out output
function YPred_test_out = LSTMnet(YPred_test)
    sig_X = [0.2380; 0.1523 ;0.0429;0.1379];
    sig_Y = 0.0690;
    mu_X = [0.0068;-0.0055;-0.0070;-0.0450];
    mu_Y = -0.0228;
    YPred_test_out = YPred_test(end);
    YPred_test_out = single(YPred_test_out* sig_Y + mu_Y)*57.3;

end

== matlab function main_RI_LIEKF_GNSSOutrage/State estimation/LI EKF2/INS propogation/AOA//SA//Vwind update/Subsystem/MATLAB Function ==
  data: u input; Rab output
function Rab = fcn(u)
    Rab = zeros(3,3);
        ca = cos(u(2));
        sa = sin(u(2));
        cb = cos(u(3));
        sb = sin(u(3));
    Rab = double([ca * cb,-ca * sb, -sa;
        sb, cb, 0;
        sa * cb, -sa * sb, ca;]);
end

== matlab function main_RI_LIEKF_GNSSOutrage/State estimation/LI EKF2/INS propogation/AOA//SA//Vwind update/Subsystem/MATLAB Function1 ==
  data: axyz input; Cl output; TAS input; alpha input
function Cl = fcn(axyz, TAS,alpha)
ax = axyz(1);
az = axyz(3);
mess = 6.9;
g = 9.79;
rou = 1.225;
a = 1.4;
b = 0.36;
S = a*b;

q = 0.5 * rou * TAS^2;

azs = -ax * sin(alpha) + az * cos(alpha);
Cl = -mess * azs / (q * S);
end

== matlab function main_RI_LIEKF_GNSSOutrage/State estimation/LI EKF2/INS propogation/AOA//SA//Vwind update/Subsystem/MATLAB Function2 ==
  data: delta input; Rbn_correct output double size=[3,3]; Rbn input
function Rbn_correct = fcn(delta, Rbn)
    delta(1) = 0;
    Rbn_correct = zeros(3,3);
     %Rbn_correct = exp_so3(delta)* Rbn;
    Rbn_correct =double(Rbn * ( eye(3) + skewMat(delta)));
end

== matlab function main_RI_LIEKF_GNSSOutrage/Sensor_Data_Process/IMU_Data_Process/gyro_preprocessing2/MATLAB Function1 ==
  data: curr_input input single; curr_output output single; sample_freq input single; cutoff_freq input single
function curr_output = second_LPF_Butter_x(curr_input,sample_freq,cutoff_freq)
   persistent input_x;
   persistent output_x;

   if isempty(input_x)
       input_x = [0;0;0];
   end
   
   if isempty(output_x)
       output_x = [0;0;0];
   end
    B = [0,0,0];
    A = [0,0,0];
    M_PI_F = 3.1415926;
	fr = sample_freq / cutoff_freq;
	ohm = tan( M_PI_F / fr );
	c = 1.0 + 2.0 * cos( M_PI_F / 4.0 ) * ohm + ohm * ohm;
	B(1) = ohm * ohm / c;
	B(2) = 2.0 * B(1);
	B(3) = B(1);
	A(1) = 2.0 * ( ohm * ohm - 1.0) / c;
	A(2) = (1.0 - 2.0 * cos( M_PI_F / 4.0 ) * ohm + ohm * ohm) / c;
	%/*获取最新输入*/
	input_x(3) = curr_input;
	%/* Butterworth */
	output_x(3) =B(1) * input_x(3) + B(2) * input_x(2) +B(3) * input_x(1) - A(1) * output_x(2) - A(2) * output_x(1);
	curr_output = single(output_x(3));
   % /* 输入序列保存 */
	input_x(1) = input_x(2);
	input_x(2) = input_x(3);
	%/*输出序列保存 */
	output_x(1) = output_x(2);
	output_x(2) = output_x(3);

== matlab function main_RI_LIEKF_GNSSOutrage/State estimation/LI EKF2/INS propogation/AOA//SA//Vwind update/Subsystem/MATLAB Function3 ==
  data: axyz input; Cy output; TAS input; alpha input; beta input
function Cy = fcn(axyz, TAS,alpha,beta)
ax = axyz(1);
ay = axyz(2);
az = axyz(3);

mess = 6.9;
g = 9.79;
rou = 1.225;
a = 1.4;
b = 0.36;
S = a*b;

q = 0.5 * rou * TAS^2;
ays = -ax .* cos(alpha).*sin(beta) + ay .* cos(beta) - az .* sin(alpha).* sin(beta);
% azs = -ax * sin(alpha) + az * cos(alpha);
Cy = mess * ays / (q * S);
end

== matlab function main_RI_LIEKF_GNSSOutrage/State estimation/LI EKF2/INS propogation/AOA//SA//Vwind update/Subsystem/MATLAB Function4 ==
  data: u input; CalculatedAttackAngleFiltered output
function CalculatedAttackAngleFiltered = fcn(u)
PitchRate = u(1);
cl = u(2);
ElevatorAngle = u(3);

coefficients_filtered = [0.0236, -0.4283, -0.0765, -0.0898];

    
CalculatedAttackAngleFiltered = (cl - ...
    coefficients_filtered(1) - ...
    coefficients_filtered(3) * PitchRate - ...
    coefficients_filtered(4) * ElevatorAngle) / coefficients_filtered(2);


end

== matlab function main_RI_LIEKF_GNSSOutrage/State estimation/LI EKF2/INS propogation/att update/MATLAB Function ==
  data: Rbn_k_1 input; Rbn output; w input; dt input
function Rbn = fcn(Rbn_k_1, w, dt)
    Rbn =  Rbn_k_1 * exp_so3( w * dt);
end

== matlab function main_RI_LIEKF_GNSSOutrage/State estimation/LI EKF2/INS propogation/att update/MATLAB Function2 ==
  data: delta input; Rbn_correct output single size=[3,3]; Rbn input
function Rbn_correct = fcn(delta, Rbn)
    Rbn_correct = zeros(3,3);
     Rbn_correct =  Rbn * exp_so3(- delta);
          % Rbn_correct = Rbn * ( eye(3) - skewMat(delta));

    %Rbn_correct =( eye(3) + skewMat(delta))* Rbn;
end

== matlab function main_RI_LIEKF_GNSSOutrage/State estimation/LI EKF2/INS propogation/vel//pos update/pos update/MATLAB Function ==
  data: dtheta input; pos_correct output single; KFState_dp input; pos input; Cbn input
function pos_correct = fcn(dtheta, KFState_dp, pos, Cbn)
    
     %pos_correct =  KFState_dp + exp_so3(dtheta)*pos;
    %pos_correct = pos + KFState_dp - skewMat(pos)*dtheta;
   pos_correct = pos + Cbn * Jl_so3(-dtheta) * KFState_dp;
   % pos_correct = pos + Cbn * KFState_dp;

end

== matlab function main_RI_LIEKF_GNSSOutrage/State estimation/LI EKF2/INS propogation/vel//pos update/vel update/MATLAB Function ==
  data: dtheta input; vel_correct output single; KFState_dv input; vel input; Cbn input
function vel_correct = fcn(dtheta, KFState_dv, vel, Cbn)
    
     %vel_correct =  KFState_dv + exp_so3( dtheta)*vel;
    %vel_correct =  vel + KFState_dv - skewMat(vel)*dtheta;
   vel_correct = vel + Cbn * Jl_so3(- dtheta) * KFState_dv;
    %vel_correct = vel + Cbn  * KFState_dv;

end

== matlab function main_RI_LIEKF_GNSSOutrage/State estimation/RI EKF_AOA_direct/INS propogation/AOA//SA//Vwind update/Subsystem/MATLAB Function1 ==
  data: dpsi input; y output
function y = wrap_dpsi(dpsi)
    if dpsi > 180
        dpsi = dpsi -360;
    elseif dpsi < -180
        dpsi = dpsi + 360;
    else 
        dpsi = dpsi;
    end
y = dpsi;

== matlab function main_RI_LIEKF_GNSSOutrage/State estimation/RI EKF_AOA_ref/Error State Kalman Filter/Cal Q1/MATLAB Function1 ==
  data: Q output; dt input
function Q = fcn(dt)
    % G.block(0, 0, 3, 3) = -exp_so3(-w_hat * dt) * Jr_so3(-w_hat * dt) * dt;
    %    G.block(6, 3, 3, 3) = -R_Gtoi.transpose() * dt;
    %    G.block(3, 3, 3, 3) = -0.5 * R_Gtoi.transpose() * dt * dt;
    %    G.block(9, 6, 3, 3).setIdentity();
    %    G.block(12, 9, 3, 3).setIdentity();
    

    cov_dim = 21;
    Q = zeros(cov_dim,cov_dim);
%     noises_sigma_a_2 = 2.0000e-4^2;
%     noises_sigma_w_2 = 1.6968e-4^2;
%     noises_sigma_ab_2 = 3.0000e-4^2;
%     noises_sigma_wb_2 = 1.9393e-5^2;
    noises_sigma_a_2 = 0.001^2*1;
    %noises_sigma_w_2 = 0.0001^2;
    noises_sigma_w_2 = 0.0001^2;
    noises_sigma_ab_2 = 1.0000e-4^2*1;
    noises_sigma_wb_2 = 0.00002^2;
    noises_sigma_mb_2 = 0.001^2;
    noises_sigma_dtheta_2 = (1/57.3)^2;
    noises_sigma_dwind_2 = 0.01^2;
    Q = diag([noises_sigma_w_2 / dt * ones(3,1); ...
                noises_sigma_a_2 / dt * ones(3,1); ...
                noises_sigma_wb_2 * dt * ones(3,1); ...
                noises_sigma_ab_2 * dt * ones(3,1); ...
                noises_sigma_mb_2 * dt * ones(3,1); ...
                noises_sigma_dtheta_2 * ones(3,1); ...
                noises_sigma_dwind_2* ones(3,1)]);
    

end

== matlab function main_RI_LIEKF_GNSSOutrage/State estimation/RI EKF_AOA_ref/Error State Kalman Filter/Extended Kalman Filter1/Correct1/Correct ==
  settings: updateMethod=DISCRETE  sampleTime=SampleTime
  data: x input; xNew output; P input; P output; yMeas input; R input; uMeas input; blockOrdering input; pM parameter; blockOrdering output
function [xNew,P,blockOrdering] = fcn(x,P,yMeas,R,uMeas,blockOrdering,pM)
% ekfCorrect Correction step for EKF
%
%   Copyright 2016-2021 The MathWorks, Inc.

%#codegen

% If measurement noise is time-varying then compute square-root
% factorization.
if pM.HasTimeVaryingR
   R = matlabshared.tracking.internal.svdPSD(R);
end

% Construct the function handle for measurement fcn
if pM.IsSimulinkFcn
    MeasurementFcnH_SL = str2func(pM.FcnName);
    if pM.HasAdditiveNoise
        MeasurementFcnH = @(fState)MeasurementFcnH_SL(fState);
    else
        MeasurementFcnH = @(fState,fMeasNoise)MeasurementFcnH_SL(fState,fMeasNoise);
    end
else
    MeasurementFcnH = str2func(pM.FcnName);
end

% Construct the function handle for measurement Jacobian fcn
if pM.HasJacobian
    if pM.IsSimulinkFcn
        MeasurementJacobianFcnH_SL = str2func(pM.JacobianFcnName);
        if pM.HasAdditiveNoise
            MeasurementJacobianFcnH = @(fState)MeasurementJacobianFcnH_SL(fState);
        else
            MeasurementJacobianFcnH = @(fState,fMeasNoise)MeasurementJacobianFcnH_SL(fState,fMeasNoise);
        end
    else
        MeasurementJacobianFcnH = str2func(pM.JacobianFcnName);
    end
else
    MeasurementJacobianFcnH = [];
end

% Handle (optional) extra input arguments of the measurement & jacobian fcns
switch pM.NumberOfExtraArgumentInports
    case 0
        extraArgs = {};
    case 1
        extraArgs = {uMeas};
    otherwise
        assert(false);
end

% Construct the corrector, perform the update
if pM.HasAdditiveNoise
    ekfCorrector = matlabshared.tracking.internal.EKFCorrectorAdditive();
else
    ekfCorrector = matlabshared.tracking.internal.EKFCorrectorNonAdditive();
end

% Check if dimensions and type of Measurement and Jacobian are correct
if pM.HasAdditiveNoise
   % Additive noise
   
   % MeasurementFcn
   ztry = MeasurementFcnH(x, extraArgs{:});
   
   if pM.IsSimulinkFcn
      hasError = (numel(ztry) ~= numel(yMeas));
   else
      hasError = (numel(ztry) ~= numel(yMeas)) || ~isa(ztry, class(x));
   end
   
   coder.internal.errorIf(...
      hasError,...
      'shared_tracking:ExtendedKalmanFilter:MeasurementNonMatchingSizeOrClass',...
      'MeasurementFcn');
   
   if pM.HasJacobian
      % MeasurementJacobianFcn
      Htry = MeasurementJacobianFcnH(x, extraArgs{:});
      isSizeNotCorrect = numel(yMeas) ~= size(Htry,1) || numel(x) ~= size(Htry,2);
      
      if pM.IsSimulinkFcn
         hasError = isSizeNotCorrect;
      else
         hasError = isSizeNotCorrect || ~isa(Htry, class(x));
      end
      
      coder.internal.errorIf(...
         hasError,...
         'shared_tracking:ExtendedKalmanFilter:MeasurementJacobianNonMatchingSizeOrClass',...
         'MeasurementJacobianFcn',numel(yMeas),numel(x));
   end   
else
   % Non-additive noise
   
   % MeasurementFcn
   ztry = MeasurementFcnH(...
      x, zeros(size(R,1),1,'like',x), ...
      extraArgs{:});   

   if pM.IsSimulinkFcn
      hasError = (numel(ztry) ~= numel(yMeas));
   else
      hasError = (numel(ztry) ~= numel(yMeas)) || ~isa(ztry, class(x));
   end
   
   coder.internal.errorIf(...
      hasError,...
      'shared_tracking:ExtendedKalmanFilter:MeasurementNonMatchingSizeOrClass',...
      'MeasurementFcn');
   
   if pM.HasJacobian
      % MeasurementJacobianFcn
      Htry = MeasurementJacobianFcnH(...
         x, zeros(size(R,1),1,'like',x), ...
         extraArgs{:});
      
      isSizeNotCorrect = numel(yMeas) ~= size(Htry,1) || numel(x) ~= size(Htry,2);     
      
      if pM.IsSimulinkFcn
         hasError = isSizeNotCorrect;
      else
         hasError = isSizeNotCorrect || ~isa(Htry, class(x));
      end
      
      coder.internal.errorIf(...
         hasError,...
         'shared_tracking:ExtendedKalmanFilter:MeasurementJacobianNonMatchingSizeOrClass',...
         'MeasurementJacobianFcn',numel(yMeas),numel(x));
   end
end
% Measurement wrapping
ekfCorrector.HasMeasurementWrapping = pM.HasWrapping;

xNew = zeros(size(x),'like',x); %#ok<PREALL>
% wk = 0;
[xNew,P] = ekfCorrector.correct(...
        yMeas,R,x,P,MeasurementFcnH,MeasurementJacobianFcnH,extraArgs{:});
end

== matlab function main_RI_LIEKF_GNSSOutrage/State estimation/RI EKF_AOA_ref/Error State Kalman Filter/Extended Kalman Filter1/Correct1/IGG_check/MATLAB Function ==
  data: err input; w output; k0 input; k1 input; zk0 input; zk1 input
function w = fcn(err,k0,k1,zk0,zk1)
    err = abs(err);  w = err;
    for k=1:2
        if err(k)<=k0,    w(k)=1;
        elseif err(k)>k1, w(k)=0;
        else,             w(k)=k0/err(k);  
        end
    end
        if err(3)<=zk0,    w(3)=1;
        elseif err(3)>zk1, w(3)=0;
        else,             w(3)=zk0/err(3);  
        end
end
